simulink model "sistema_lti_simplificado"  (R2019a)
settings: Solver=ode45  StartTime=0.0  StopTime=10.0  MaxStep=1e-6  RelTol=1e-6
undefined symbols (not defined in the file): b_eq, dT_l, J_eq, L_q, lambda_m, P_p, r, R_s_prom
libraries: simulink x2, eeTransforms x1
settings Model: Creator=pedro  LastModifiedBy=pedro

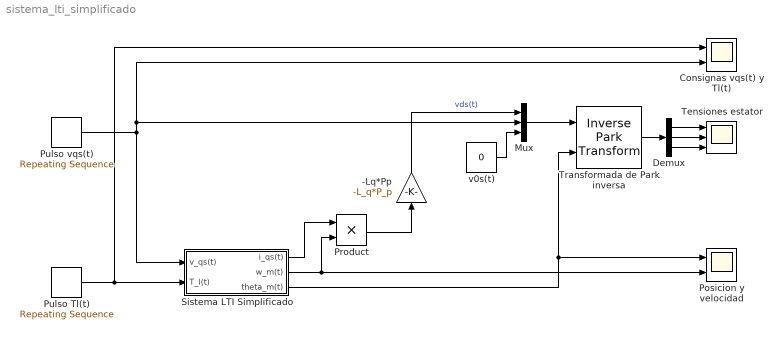
== system sistema_lti_simplificado ==
  -Lq*Pp : Gain  Gain=-L_q*P_p
  Consignas vqs(t) y Tl(t) : Scope  NumInputPorts=2
  Demux : Demux  Outputs=3
  Mux : Mux  Inputs=3
  Posicion y velocidad : Scope  NumInputPorts=2
  Product : Product
  Pulso Tl(t) : simulink/Sources/Repeating Sequence  rep_seq_t=[0 0.299 0.3 0.499 0.5 0.899 0.9 10]  rep_seq_y=[0 0 dT_l dT_l -dT_l -dT_l 0 0]
  Pulso vqs(t) : simulink/Sources/Repeating Sequence  rep_seq_t=[0 0.099 0.1 0.699 0.7 10]  rep_seq_y=[0 0 19.596 19.596 0 0]
  Sistema LTI Simplificado : Subsystem
  Tensiones estator : Scope  NumInputPorts=3
  "Transformada de Park inversa " : eeTransforms/Inverse Park Transform  AxisAlignment=Q-axis  PowerInvariant=off
      settings: SourceProductName=Simscape Electrical
  v0s(t) : Constant  Value=0
  wires:
  Pulso Tl(t)/1 -> Consignas vqs(t) y Tl(t)/1, Sistema LTI Simplificado/2("T_l(t) ")
  Demux/3 -> Tensiones estator/3
  Sistema LTI Simplificado/2(w_m(t)) -> Product/2, Posicion y velocidad/2
  v0s(t)/1 -> Mux/3
  "Transformada de Park inversa "/1 -> Demux/1
  Sistema LTI Simplificado/3(theta_m(t)) -> Posicion y velocidad/1, "Transformada de Park inversa "/2
  Mux/1 -> "Transformada de Park inversa "/1
  Pulso vqs(t)/1 -> Consignas vqs(t) y Tl(t)/2, Mux/2, Sistema LTI Simplificado/1(v_qs(t))
  Demux/1 -> Tensiones estator/1
  Demux/2 -> Tensiones estator/2
  Sistema LTI Simplificado/1("i_qs(t) ") -> Product/1
  Product/1 -> -Lq*Pp/1
  -Lq*Pp/1 -> Mux/1  "vds(t)"

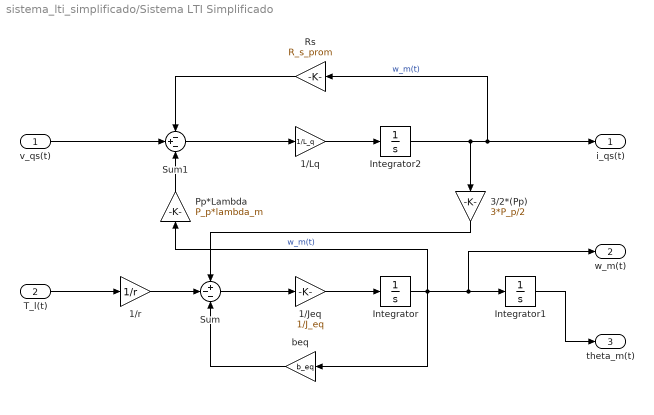
== system sistema_lti_simplificado/Sistema LTI Simplificado ==
  v_qs(t) : Inport
  "T_l(t) " : Inport  Port=2
  "1/Jeq " : Gain  Gain=1/J_eq
  1/Lq : Gain  Gain=1/L_q
  1/r : Gain  Gain=1/r
  3/2*(Pp) : Gain  Gain=3*P_p/2
  Integrator : Integrator
  Integrator1 : Integrator
  Integrator2 : Integrator
  Pp*Lambda : Gain  Gain=P_p*lambda_m
  Rs : Gain  Gain=R_s_prom
  Sum : Sum  Inputs=+--
  Sum1 : Sum  Inputs=-+-
  beq : Gain  Gain=b_eq
  "i_qs(t) " : Outport
  w_m(t) : Outport  Port=2
  theta_m(t) : Outport  Port=3
  wires:
  1/r/1 -> Sum/2
  "T_l(t) "/1 -> 1/r/1
  Sum/1 -> "1/Jeq "/1
  "1/Jeq "/1 -> Integrator/1
  Integrator/1 -> Pp*Lambda/1, beq/1, w_m(t)/1, Integrator1/1  "w_m(t)"
  beq/1 -> Sum/3
  v_qs(t)/1 -> Sum1/2
  Sum1/1 -> 1/Lq/1
  Pp*Lambda/1 -> Sum1/3
  1/Lq/1 -> Integrator2/1
  Integrator2/1 -> Rs/1, "i_qs(t) "/1, 3/2*(Pp)/1  "w_m(t)"
  Rs/1 -> Sum1/1
  3/2*(Pp)/1 -> Sum/1
  Integrator1/1 -> theta_m(t)/1
